simulink model "ex8imp"  (R2025b)
settings: Solver=VariableStepAuto  StartTime=0.0  StopTime=Tfin  RelTol=1e-3
values from neighbouring files (symbols this model uses):
  x0 = [rand,rand]    [ex2.m]    (also in ex3.m = [randi([-5,5]),randi([-5,5]),randi([0,5])]; ex8.m = [0;0;0])
settings Model: Creator=Esteban  LastModifiedBy=Esteban

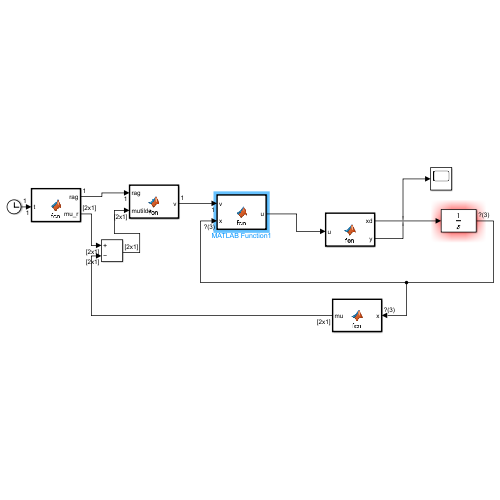
[thumbnail: Simulink's stored preview of the top-level diagram]
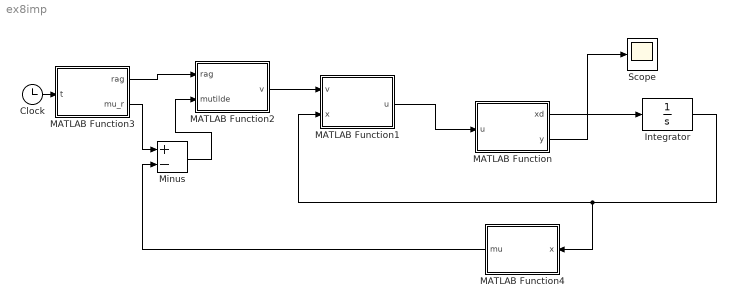
== system ex8imp ==
  Clock : Clock
  Integrator : Integrator  InitialCondition=x0
  MATLAB Function : MATLAB Function  TreatAsAtomicUnit=on
  MATLAB Function1 : MATLAB Function  TreatAsAtomicUnit=on
  MATLAB Function2 : MATLAB Function  TreatAsAtomicUnit=on
  MATLAB Function3 : MATLAB Function  TreatAsAtomicUnit=on
  MATLAB Function4 : MATLAB Function  TreatAsAtomicUnit=on
  Minus : Sum  Inputs=+-
  Scope : Scope
  wires:
  MATLAB Function/1(xd) -> Integrator/1
  MATLAB Function1/1(u) -> MATLAB Function/1(u)
  MATLAB Function2/1(v) -> MATLAB Function1/1(v)
  Integrator/1 -> MATLAB Function4/1(x), MATLAB Function1/2(x)
  MATLAB Function/2(y) -> Scope/1
  Clock/1 -> MATLAB Function3/1(t)
  MATLAB Function3/1(rag) -> MATLAB Function2/1(rag)
  MATLAB Function4/1(mu) -> Minus/2
  MATLAB Function3/2(mu_r) -> Minus/1
  Minus/1 -> MATLAB Function2/2(mutilde)

== matlab function ex8imp/MATLAB Function ==
  data: u input; xd output; y output
function [xd,y] = fcn(u)
a = 10.82;
b = 14.286;
R = 0.01;
c1 = 1.3;
c2 = 0.22;
ro =  -c2*sin(pi*x(1)/c1);
xd = zeros(3,1);
xd(1,:) = a*(x(2)-ro);
xd(2,:) = x(1) - x(2) + x(3) + u;
xd(3,:) = -b*x(2) - R*x(3);

y = x(1);

== matlab function ex8imp/MATLAB Function2 ==
  data: rag input; v output; mutilde input
function v = fcn(rag, mutilde)


k1 = 50;
k2 = 30;

n = 5;

s = k2*mutilde(1);
v = rag + k2*mutilde(1)+k1*tanh(n*s);

== matlab function ex8imp/MATLAB Function3 ==
  data: rag output; t input; mu_r output
function [rag,mu_r] = fcn(t)

r = sin(t);

rag = cos(t);

mu_r = [r;rag];

== matlab function ex8imp/MATLAB Function4 ==
  data: x input; mu output
function mu = fcn(x)
c1 = 1.3;
c2 = 0.22;
ro =  -c2*sin(pi*x(1)/c1);
mu = zeros(2,1);
mu = [x(1);a*(x(2)-ro)];

== matlab function ex8imp/MATLAB Function1 ==
  data: v input; x input; u output
function u = fcn(v, x)
a = 10.82;
c1 = 1.3;
c2 = 0.22;
ro =  -c2*sin(pi*x(1)/c1);

u = 1/a *(x(1)+x(2)-x(3)+v-diff(ro)*(a*(x(2)-ro)));
